simulink model "Exemplu_figura7"  (R2016a)
settings: Solver=VariableStepDiscrete  StartTime=0.0  StopTime=10.0  RelTol=1e-3
settings Model: Creator=Cristina  LastModifiedBy=Cristina

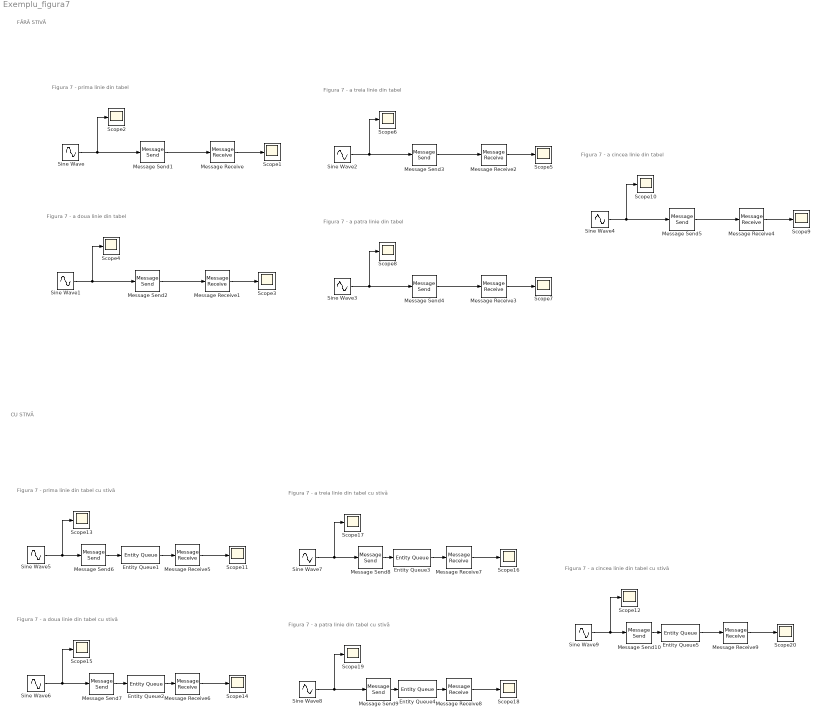
== system Exemplu_figura7 ==
  note: CU STIVĂ
  note: FĂRĂ STIVĂ
  note: Figura 7 - prima linie din tabel
  note: Figura 7 - a doua linie din tabel
  note: Figura 7 - a treia linie din tabel
  note: Figura 7 - a patra linie din tabel
  note: Figura 7 - a cincea linie din tabel
  note: Figura 7 - prima linie din tabel cu stivă
  note: Figura 7 - a doua linie din tabel cu stivă
  note: Figura 7 - a treia linie din tabel cu stivă
  note: Figura 7 - a patra linie din tabel cu stivă
  note: Figura 7 - a cincea linie din tabel cu stivă
  Entity Queue{1..5} (5 alike) : EntityQueue  InputPortMessageModes=m  OutputPortMessageModes=m
      settings: OutputPortMap=o5
  Message Receive{,4..5,9} (4 alike) : MessageReceive  InputPortMessageModes=m  SampleTime=0.1
      settings: OutputPortMap=o1
  Message Receive{1,3,6,8} (4 alike) : MessageReceive  InputPortMessageModes=m  SampleTime=0.2
      settings: OutputPortMap=o1
  Message Receive2 : MessageReceive  InputPortMessageModes=m  QueueLength=32  SampleTime=0.2
      settings: OutputPortMap=o1
  Message Receive7 : MessageReceive  InputPortMessageModes=m  QueueLength=32  SampleTime=0.2
      settings: OutputPortMap=o1
  Message Send{1..10} (10 alike) : MessageSend  OutputPortMessageModes=m
      settings: InputPortMap=u1
  Scope{1..20} (20 alike) : Scope
  Sine Wave{,1..2,5..7} (6 alike) : Sin  SampleTime=0.1
  Sine Wave{3..4,8..9} (4 alike) : Sin  SampleTime=0.2
  wires:
  Sine Wave/1 -> Scope2/1, Message Send1/1
  Message Send1/1 -> Message Receive/1
  Message Receive/1 -> Scope1/1
  Sine Wave1/1 -> Message Send2/1, Scope4/1
  Message Send2/1 -> Message Receive1/1
  Message Receive1/1 -> Scope3/1
  Sine Wave2/1 -> Message Send3/1, Scope6/1
  Message Send3/1 -> Message Receive2/1
  Message Receive2/1 -> Scope5/1
  Sine Wave3/1 -> Message Send4/1, Scope8/1
  Message Send4/1 -> Message Receive3/1
  Message Receive3/1 -> Scope7/1
  Sine Wave4/1 -> Message Send5/1, Scope10/1
  Message Send5/1 -> Message Receive4/1
  Message Receive4/1 -> Scope9/1
  Sine Wave5/1 -> Scope13/1, Message Send6/1
  Message Send6/1 -> Entity Queue1/1
  Message Receive5/1 -> Scope11/1
  Sine Wave6/1 -> Message Send7/1, Scope15/1
  Message Send7/1 -> Entity Queue2/1
  Message Receive6/1 -> Scope14/1
  Sine Wave7/1 -> Message Send8/1, Scope17/1
  Message Send8/1 -> Entity Queue3/1
  Message Receive7/1 -> Scope16/1
  Sine Wave8/1 -> Message Send9/1, Scope19/1
  Message Receive8/1 -> Scope18/1
  Sine Wave9/1 -> Message Send10/1, Scope12/1
  Message Send10/1 -> Entity Queue5/1
  Message Receive9/1 -> Scope20/1
  Entity Queue1/1 -> Message Receive5/1
  Entity Queue2/1 -> Message Receive6/1
  Entity Queue3/1 -> Message Receive7/1
  Message Send9/1 -> Entity Queue4/1
  Entity Queue4/1 -> Message Receive8/1
  Entity Queue5/1 -> Message Receive9/1
